simulink library "marine_gnc"  (Simulink 7.4)
settings: Solver=ode45  SolverMode=SingleTasking  StartTime=0.0  StopTime=10.0  RelTol=1e-3
undefined symbols (not defined in the file or in its folder): CN_data, CX_data, CY_data, D, G, K_supply, kt2ms, M, MA, magnitude, marine, Models, MRB, order, pathlength, RAO_Amp, RAO_Dir, RAO_Freq, RAO_Phase, RAO_Vel, RAO_yaw_back, RAO_yaw_quant, RAO_yaw_quantization_flag, rho_a, Semi, sub, T_supply, table, Tanker, vessel, Vessels
libraries: marine_gnc x64, simulink x39, cybersealib x1
(part 5 of 6)

== system marine_gnc/Utilities/Math Operations/[-inf inf] to [-pi pi] ==
  note: r
  note: x
  x [-inf inf] : Inport  OutDataType=sfix(16)  OutScaling=2^0
  Constant : Constant  Value=2*pi  OutDataType=sfix(16)  OutScaling=2^0
  Gain : Gain  Gain=pi  ParameterDataType=sfix(16)  ParameterScaling=2^0  OutDataType=sfix(16)  OutScaling=2^0  SaturateOnIntegerOverflow=on  OutDataTypeStr=Inherit: Same as input  ParamDataTypeStr=Inherit: Same as input
  Math Function : Math  Operator=rem  OutDataType=sfix(16)  OutScaling=2^0  SaturateOnIntegerOverflow=on
  Saturation : Saturate  UpperLimit=1e10  LowerLimit=-1e10
  Sign : Signum
  Sum : Sum  Inputs=|+-  OutDataType=sfix(16)  OutScaling=2^0  SaturateOnIntegerOverflow=on
  Sum1 : Sum  Inputs=|++  OutDataType=sfix(16)  OutScaling=2^0  SaturateOnIntegerOverflow=on
  y [-pi pi] : Outport  OutDataType=sfix(16)  OutScaling=2^0
  wires:
  Saturation/1 -> Sign/1, Sum1/1
  Sum/1 -> y [-pi pi]/1
  Math Function/1 -> Sum/1
  Constant/1 -> Math Function/2
  Sum1/1 -> Math Function/1
  Gain/1 -> Sum1/2, Sum/2
  Sign/1 -> Gain/1
  x [-inf inf]/1 -> Saturation/1

== system marine_gnc/Utilities/Math Operations/[-pi pi] to [-inf inf] ==
  x [-pi pi] : Inport  OutDataType=sfix(16)  OutScaling=2^0
  S-Function : S-Function  FunctionName=pipi2inf  EnableBusSupport=off
  y [-inf inf] : Outport  OutDataType=sfix(16)  OutScaling=2^0
  wires:
  S-Function/1 -> y [-inf inf]/1
  x [-pi pi]/1 -> S-Function/1

== system marine_gnc/Utilities/Math Operations/deg to 180/180 ==
  note: r
  note: x
  x (deg) : Inport  OutDataType=sfix(16)  OutScaling=2^0
  Constant : Constant  Value=2*180  OutDataType=sfix(16)  OutScaling=2^0
  Gain : Gain  Gain=180  ParameterDataType=sfix(16)  ParameterScaling=2^0  OutDataType=sfix(16)  OutScaling=2^0  SaturateOnIntegerOverflow=on  OutDataTypeStr=Inherit: Same as input  ParamDataTypeStr=Inherit: Same as input
  Math Function : Math  Operator=rem  OutDataType=sfix(16)  OutScaling=2^0  SaturateOnIntegerOverflow=on
  Saturation : Saturate  UpperLimit=1e10  LowerLimit=-1e10
  Sign : Signum
  Sum : Sum  Inputs=|+-  OutDataType=sfix(16)  OutScaling=2^0  SaturateOnIntegerOverflow=on
  Sum1 : Sum  Inputs=|++  OutDataType=sfix(16)  OutScaling=2^0  SaturateOnIntegerOverflow=on
  -180<y<180 : Outport  OutDataType=sfix(16)  OutScaling=2^0
  wires:
  Sum/1 -> -180<y<180/1
  Math Function/1 -> Sum/1
  Constant/1 -> Math Function/2
  Sum1/1 -> Math Function/1
  Gain/1 -> Sum1/2, Sum/2
  Sign/1 -> Gain/1
  x (deg)/1 -> Saturation/1
  Saturation/1 -> Sign/1, Sum1/1

== system marine_gnc/Utilities/Simulation tools/6DOF comparison ==
  In 1 : Inport  OutDataType=sfix(16)  OutScaling=2^0
  In 2 : Inport  Port=2  OutDataType=sfix(16)  OutScaling=2^0
  6DOF comparison : Scope  NumInputPorts=6
      settings: TimeRange=200  YMin=-0.2~-0.15~-0.5~-0.2~-0.02~-0.015  YMax=0.3~0.175~0.5~0.2~0.02~0.0175  MaxDataPoints=20000
  Demux1 : Demux  Outputs=6
  Demux2 : Demux  Outputs=6
  Mux{,1..5} (6 alike) : Mux  Inputs=2
  wires:
  Demux2/1 -> Mux/1  "surge"
  Demux1/1 -> Mux/2  "surge"
  Demux2/2 -> Mux1/1  "sway"
  Demux2/3 -> Mux2/1  "heave"
  Demux2/4 -> Mux3/1  "roll"
  Demux2/5 -> Mux4/1  "pitch"
  Demux2/6 -> Mux5/1  "yaw"
  Demux1/2 -> Mux1/2
  Demux1/3 -> Mux2/2
  Demux1/4 -> Mux3/2
  Demux1/5 -> Mux4/2
  Demux1/6 -> Mux5/2
  In 1/1 -> Demux2/1
  In 2/1 -> Demux1/1
  Mux/1 -> 6DOF comparison/1  "surge"
  Mux1/1 -> 6DOF comparison/2  "sway"
  Mux2/1 -> 6DOF comparison/3  "heave"
  Mux3/1 -> 6DOF comparison/4  "roll"
  Mux4/1 -> 6DOF comparison/5  "pitch"
  Mux5/1 -> 6DOF comparison/6  "yaw"

== system marine_gnc/Utilities/Simulation tools/Signal range error ==
  Signal : Inport  OutDataType=sfix(16)  OutScaling=2^0
  Add : Sum  OutDataType=sfix(16)  OutScaling=2^-10
  Constant : Constant  Value=Values  OutDataType=sfix(16)  OutScaling=2^0
  MinMax : MinMax  Function=max  OutDataType=sfix(16)  OutScaling=2^0
  MinMax1 : MinMax  Function=max  OutDataType=sfix(16)  OutScaling=2^0
  MinMax2 : MinMax  OutDataType=sfix(16)  OutScaling=2^0
  MinMax3 : MinMax  OutDataType=sfix(16)  OutScaling=2^0
  Saturation : Saturate  UpperLimit=1  LowerLimit=0
  Saturation1 : Saturate  UpperLimit=1  LowerLimit=0
  Sign : Signum
  Sign1 : Signum
  Stop simulation : marine_gnc/Utilities/Simulation tools/Stop simulation  message=message
  Subtract : Sum  Inputs=+-  OutDataType=sfix(16)  OutScaling=2^-10
  Subtract1 : Sum  Inputs=-+  OutDataType=sfix(16)  OutScaling=2^-10
  wires:
  Sign/1 -> Saturation/1
  Signal/1 -> MinMax/1, MinMax2/1
  Constant/1 -> MinMax1/1, MinMax3/1
  MinMax/1 -> Subtract/1
  MinMax1/1 -> Subtract/2
  Subtract/1 -> Sign/1
  Saturation/1 -> Add/1
  Add/1 -> Stop simulation/1
  Sign1/1 -> Saturation1/1
  Subtract1/1 -> Sign1/1
  MinMax2/1 -> Subtract1/1
  MinMax3/1 -> Subtract1/2
  Saturation1/1 -> Add/2

== system marine_gnc/Environment/Wind/Wind/Slowly-varying wind ==
  Enable : EnablePort
  Band-Limited White Noise : simulink/Sources/Band-Limited White Noise  Cov=Par_Wind_speed_noise_pow  Ts=Par_Wind_sample_time  seed=Par_Wind_speed_seed
  "Band-Limited White Noise " : simulink/Sources/Band-Limited White Noise  Cov=Par_Wind_angle_noise_pow  Ts=Par_Wind_sample_time  seed=Par_Wind_angle_seed
  Gain : Gain  Gain=1/Par_Wind_speed_T  ParameterDataType=sfix(16)  ParameterScaling=2^0  OutDataType=sfix(16)  OutScaling=2^0  SaturateOnIntegerOverflow=on  OutDataTypeStr=Inherit: Same as input  ParamDataTypeStr=Inherit: Same as input
  "Gain " : Gain  Gain=1/Par_Wind_angle_T  ParameterDataType=sfix(16)  ParameterScaling=2^0  OutDataType=sfix(16)  OutScaling=2^0  SaturateOnIntegerOverflow=on  OutDataTypeStr=Inherit: Same as input  ParamDataTypeStr=Inherit: Same as input
  Integrator : Integrator  LimitOutput=on  UpperSaturationLimit=Par_Wind_speed_rand_max  LowerSaturationLimit=-Par_Wind_speed_rand_max
  "Integrator " : Integrator  LimitOutput=on  UpperSaturationLimit=Par_Wind_angle_rand_max  LowerSaturationLimit=-Par_Wind_angle_rand_max
  Sum : Sum  Inputs=|+-  OutDataType=sfix(16)  OutScaling=2^0  SaturateOnIntegerOverflow=on  InputSameDT=on  OutDataTypeStr=Inherit: Same as first input
  "Sum       " : Sum  Inputs=|+-  OutDataType=sfix(16)  OutScaling=2^0  SaturateOnIntegerOverflow=on  InputSameDT=on  OutDataTypeStr=Inherit: Same as first input
  angle : Outport  OutDataType=sfix(16)  OutScaling=2^0  InitialOutput=0
  speed : Outport  Port=2  OutDataType=sfix(16)  OutScaling=2^0  InitialOutput=0
  wires:
  Band-Limited White Noise/1 -> Sum/1
  Integrator/1 -> Sum/2, speed/1
  Sum/1 -> Gain/1
  Gain/1 -> Integrator/1
  "Band-Limited White Noise "/1 -> "Sum       "/1
  "Integrator "/1 -> "Sum       "/2, angle/1
  "Sum       "/1 -> "Gain "/1
  "Gain "/1 -> "Integrator "/1

== system marine_gnc/Environment/Wind/Wind/Wind gust ==
  u10 : Inport  OutDataType=sfix(16)  OutScaling=2^0
  Enable : EnablePort
  Clock : Clock
      settings: Decimation=10
  Dot Product : simulink/Math Operations/Dot Product  InputSameDT=on  OutDataType=sfix(16)  OutScaling=2^-10  DoSatur=off
  Frequencies : Constant  Value=Par_Wind_minfreq:(Par_Wind_maxfreq - Par_Wind_minfreq)/(Par_Wind_nfreq-1):Par_Wind_maxfreq  OutDataType=sfix(16)  OutScaling=2^0
  Gain : Gain  Gain=2  ParameterDataType=sfix(16)  ParameterScaling=2^0  OutDataType=sfix(16)  OutScaling=2^0  SaturateOnIntegerOverflow=on  OutDataTypeStr=Inherit: Same as input  ParamDataTypeStr=Inherit: Same as input
  Gain1 : Gain  Gain=2*pi  ParameterDataType=sfix(16)  ParameterScaling=2^0  OutDataType=sfix(16)  OutScaling=2^0  SaturateOnIntegerOverflow=on  OutDataTypeStr=Inherit: Same as input  ParamDataTypeStr=Inherit: Same as input
  Harris spectrum : Subsystem
  Math Function1 : Math  Operator=sqrt  OutDataType=sfix(16)  OutScaling=2^0  SaturateOnIntegerOverflow=on
  Multiport Switch : MultiPortSwitch  Inputs=2  RndMeth=Nearest  SaturateOnIntegerOverflow=on
  NORSOK spectrum : Subsystem
  Phase generator : Subsystem
  Product1 : Product  OutDataType=sfix(16)  OutScaling=2^0  SaturateOnIntegerOverflow=on  OutDataTypeStr=Inherit: Same as first input
  Product2 : Product  OutDataType=sfix(16)  OutScaling=2^0  SaturateOnIntegerOverflow=on  OutDataTypeStr=Inherit: Same as first input
  Saturation : Saturate  UpperLimit=2  LowerLimit=1
  Spectrum type : Constant  Value=Par_Wind_spectrum_type  OutDataType=sfix(16)  OutScaling=2^0
  Sum : Sum  OutDataType=sfix(16)  OutScaling=2^0  SaturateOnIntegerOverflow=on
  Trigonometric Function : Trigonometry
  dfreq : Constant  Value=(Par_Wind_maxfreq - Par_Wind_minfreq)/(Par_Wind_nfreq -1)  OutDataType=sfix(16)  OutScaling=2^0
  Gust : Outport  OutDataType=sfix(16)  OutScaling=2^0  InitialOutput=0
  wires:
  Saturation/1 -> Multiport Switch/1
  Frequencies/1 -> Harris spectrum/1(Freqs), NORSOK spectrum/1(Freqs), Gain1/1
  u10/1 -> NORSOK spectrum/2(u10), Harris spectrum/2(u10)
  Gain/1 -> Product1/1
  dfreq/1 -> Product1/2
  Product1/1 -> Math Function1/1
  Multiport Switch/1 -> Gain/1
  Spectrum type/1 -> Saturation/1
  Harris spectrum/1(S) -> Multiport Switch/2
  NORSOK spectrum/1(S) -> Multiport Switch/3
  Gain1/1 -> Product2/1
  Clock/1 -> Product2/2, Phase generator/Trigger
  Product2/1 -> Sum/1  "wt"
  Phase generator/1(Phase) -> Sum/2
  Sum/1 -> Trigonometric Function/1
  Math Function1/1 -> Dot Product/1  "Amp"
  Trigonometric Function/1 -> Dot Product/2  "sin(wt + phase)"
  Dot Product/1 -> Gust/1

== system marine_gnc/Examples/Vessels/CyberShipII/saturation ==
  tau : Inport  OutDataType=sfix(16)  OutScaling=2^0
  Demux : Demux  Outputs=3
  Mux1 : Mux  Inputs=3
  Saturation : Saturate  UpperLimit=2  LowerLimit=-2
  Saturation1 : Saturate  UpperLimit=1.5  LowerLimit=-1.5
  Saturation2 : Saturate  UpperLimit=1.5  LowerLimit=-1.5
  sat_tau : Outport  OutDataType=sfix(16)  OutScaling=2^0
  wires:
  Mux1/1 -> sat_tau/1
  tau/1 -> Demux/1
  Demux/1 -> Saturation/1
  Demux/2 -> Saturation1/1
  Demux/3 -> Saturation2/1
  Saturation/1 -> Mux1/1
  Saturation1/1 -> Mux1/2
  Saturation2/1 -> Mux1/3

== system marine_gnc/Examples/Vessels/Mariner class cargo ship  (2nd -order)/Ship model ==
  note: heading
      | angle
  rudder angle : Inport  OutDataType=sfix(16)  OutScaling=2^0
  Integrator : Integrator
  Nomoto 2nd-order model : TransferFcn  Numerator=[K*T3 K]  Denominator=[T1*T2 (T1+T2) 1]
  heading angle : Outport  OutDataType=sfix(16)  OutScaling=2^0
  heading rate : Outport  Port=2  OutDataType=sfix(16)  OutScaling=2^0
  wires:
  rudder angle/1 -> Nomoto 2nd-order model/1
  Nomoto 2nd-order model/1 -> heading rate/1, Integrator/1  "heading rate"
  Integrator/1 -> heading angle/1

== system marine_gnc/Examples/Vessels/Tanker (1st-order)/Ship model ==
  note: heading
      | angle
  rudder angle : Inport  OutDataType=sfix(16)  OutScaling=2^0
  " Nomoto  time constant" : Gain  Gain=1/T_supply  ParameterDataType=sfix(16)  ParameterScaling=2^0  OutDataType=sfix(16)  OutScaling=2^0  SaturateOnIntegerOverflow=on  OutDataTypeStr=Inherit: Same as input  ParamDataTypeStr=Inherit: Same as input
  Integrator : Integrator
  Integrator1 : Integrator
  Nomoto gain constant : Gain  Gain=K_supply  ParameterDataType=sfix(16)  ParameterScaling=2^0  OutDataType=sfix(16)  OutScaling=2^0  SaturateOnIntegerOverflow=on  OutDataTypeStr=Inherit: Same as input  ParamDataTypeStr=Inherit: Same as input
  Sum : Sum  Inputs=|+-  OutDataType=sfix(16)  OutScaling=2^0  SaturateOnIntegerOverflow=on  InputSameDT=on  OutDataTypeStr=Inherit: Same as first input
  heading angle : Outport  OutDataType=sfix(16)  OutScaling=2^0
  heading rate : Outport  Port=2  OutDataType=sfix(16)  OutScaling=2^0
  wires:
  Integrator1/1 -> heading angle/1
  Integrator/1 -> Sum/2, Integrator1/1, heading rate/1  "heading  rate"
  Nomoto gain constant/1 -> Sum/1
  rudder angle/1 -> Nomoto gain constant/1
  Sum/1 -> " Nomoto  time constant"/1
  " Nomoto  time constant"/1 -> Integrator/1

== system marine_gnc/Examples/Vessels/Tanker (2nd-order)/Ship model ==
  note: heading
      | angle
  rudder angle : Inport  OutDataType=sfix(16)  OutScaling=2^0
  Integrator : Integrator
  Nomoto 2nd-order model : TransferFcn  Numerator=[K*T3 K]  Denominator=[T1*T2 (T1+T2) 1]
  heading angle : Outport  OutDataType=sfix(16)  OutScaling=2^0
  heading rate : Outport  Port=2  OutDataType=sfix(16)  OutScaling=2^0
  wires:
  rudder angle/1 -> Nomoto 2nd-order model/1
  Nomoto 2nd-order model/1 -> heading rate/1, Integrator/1  "heading rate"
  Integrator/1 -> heading angle/1

== system marine_gnc/Examples/Vessels/m-file examples/Container ship: L = 175 m ==
  u : Inport  OutDataType=sfix(16)  OutScaling=2^0
  xo : Inport  Port=2  OutDataType=sfix(16)  OutScaling=2^0
  Integrator : Integrator  InitialConditionSource=external  InitialCondition=[1 1]  UpperSaturationLimit=10  LowerSaturationLimit=-10
  Mux1 : Mux  Inputs=2
  m-file : MATLABFcn  MATLABFcn=feval(vessmodel,u(1:dimx_model),u(dimx_model+1:length(u)))  Output1D=off
  x : Outport  OutDataType=sfix(16)  OutScaling=2^0
  wires:
  xo/1 -> Integrator/2
  u/1 -> Mux1/2
  Mux1/1 -> m-file/1
  Integrator/1 -> x/1, Mux1/1
  m-file/1 -> Integrator/1

== system marine_gnc/Examples/Vessels/m-file examples/Deep submergence rescue vehicle ==
  u : Inport  OutDataType=sfix(16)  OutScaling=2^0
  xo : Inport  Port=2  OutDataType=sfix(16)  OutScaling=2^0
  Integrator : Integrator  InitialConditionSource=external  InitialCondition=[1 1]  UpperSaturationLimit=10  LowerSaturationLimit=-10
  Mux1 : Mux  Inputs=2
  m-file : MATLABFcn  MATLABFcn=feval(vessmodel,u(1:dimx_model),u(dimx_model+1:length(u)))  Output1D=off
  x : Outport  OutDataType=sfix(16)  OutScaling=2^0
  wires:
  xo/1 -> Integrator/2
  u/1 -> Mux1/2
  Mux1/1 -> m-file/1
  Integrator/1 -> x/1, Mux1/1
  m-file/1 -> Integrator/1

== system marine_gnc/Examples/Vessels/m-file examples/Large tanker: L = 304 m ==
  u : Inport  OutDataType=sfix(16)  OutScaling=2^0
  xo : Inport  Port=2  OutDataType=sfix(16)  OutScaling=2^0
  Integrator : Integrator  InitialConditionSource=external  InitialCondition=[1 1]  UpperSaturationLimit=10  LowerSaturationLimit=-10
  Mux1 : Mux  Inputs=2
  m-file : MATLABFcn  MATLABFcn=feval(vessmodel,u(1:dimx_model),u(dimx_model+1:length(u)))  Output1D=off
  x : Outport  OutDataType=sfix(16)  OutScaling=2^0
  wires:
  xo/1 -> Integrator/2
  u/1 -> Mux1/2
  Mux1/1 -> m-file/1
  Integrator/1 -> x/1, Mux1/1
  m-file/1 -> Integrator/1

== system marine_gnc/Examples/Vessels/m-file examples/Mariner class vessel: L = 160 m ==
  u : Inport  OutDataType=sfix(16)  OutScaling=2^0
  xo : Inport  Port=2  OutDataType=sfix(16)  OutScaling=2^0
  Integrator : Integrator  InitialConditionSource=external  InitialCondition=[1 1]  UpperSaturationLimit=10  LowerSaturationLimit=-10
  Mux1 : Mux  Inputs=2
  m-file : MATLABFcn  MATLABFcn=feval(vessmodel,u(1:dimx_model),u(dimx_model+1:length(u)))  Output1D=off
  x : Outport  OutDataType=sfix(16)  OutScaling=2^0
  wires:
  xo/1 -> Integrator/2
  u/1 -> Mux1/2
  Mux1/1 -> m-file/1
  Integrator/1 -> x/1, Mux1/1
  m-file/1 -> Integrator/1

== system marine_gnc/Examples/Vessels/m-file examples/Naval Postgraduate School AUV ==
  u : Inport  OutDataType=sfix(16)  OutScaling=2^0
  xo : Inport  Port=2  OutDataType=sfix(16)  OutScaling=2^0
  Integrator : Integrator  InitialConditionSource=external  InitialCondition=[1 1]  UpperSaturationLimit=10  LowerSaturationLimit=-10
  Mux1 : Mux  Inputs=2
  m-file : MATLABFcn  MATLABFcn=feval(vessmodel,u(1:dimx_model),u(dimx_model+1:length(u)))  Output1D=off
  x : Outport  OutDataType=sfix(16)  OutScaling=2^0
  wires:
  xo/1 -> Integrator/2
  u/1 -> Mux1/2
  Mux1/1 -> m-file/1
  Integrator/1 -> x/1, Mux1/1
  m-file/1 -> Integrator/1

== system marine_gnc/Guidance/Way-point guidance block/Stop vessel/Reached endpoint ==
  IfAction : ActionPort
  Constant : Constant  Value=0  OutDataType=sfix(16)  OutScaling=2^0
  Stop Simulation : Stop
  stop : Constant  Value=stop  OutDataType=sfix(16)  OutScaling=2^0
  zero : Outport  OutDataType=sfix(16)  OutScaling=2^0
  wires:
  Constant/1 -> zero/1
  stop/1 -> Stop Simulation/1

== system marine_gnc/Guidance/Way-point guidance block/Stop vessel/Still travelling ==
  IfAction : ActionPort
  Constant : Constant  OutDataType=sfix(16)  OutScaling=2^0
  one : Outport  OutDataType=sfix(16)  OutScaling=2^0
  wires:
  Constant/1 -> one/1

== system marine_gnc/Guidance/Way-point guidance block/Thetacomputation/5th order algorithm ==
  theta : Inport  OutDataType=sfix(16)  OutScaling=2^0
  IfAction : ActionPort
  Constant1 : Constant  OutDataType=sfix(16)  OutScaling=2^0
  Constant2 : Constant  OutDataType=sfix(16)  OutScaling=2^0
  Math Function : Math  Operator=mod  OutDataType=sfix(16)  OutScaling=2^0  SaturateOnIntegerOverflow=on
  Mux1 : Mux  Inputs=6
  Product{,1..3} (4 alike) : Product  OutDataType=sfix(16)  OutScaling=2^0  SaturateOnIntegerOverflow=on  InputSameDT=on  OutDataTypeStr=Inherit: Same as first input
  theta_vector : Outport  OutDataType=sfix(16)  OutScaling=2^0
  wires:
  Constant1/1 -> Math Function/2
  Math Function/1 -> Product/1, Product1/2, Product2/2, Product3/2, Mux1/5, Product/2
  theta/1 -> Math Function/1
  Product/1 -> Product1/1, Mux1/4  "t^2"
  Product1/1 -> Product2/1, Mux1/3  "t^3"
  Product2/1 -> Mux1/2, Product3/1  "t^4"
  Product3/1 -> Mux1/1
  Constant2/1 -> Mux1/6
  Mux1/1 -> theta_vector/1

== system marine_gnc/Guidance/Way-point guidance block/Thetacomputation/Cubic splines ==
  theta : Inport  OutDataType=sfix(16)  OutScaling=2^0
  IfAction : ActionPort
  Constant1 : Constant  OutDataType=sfix(16)  OutScaling=2^0
  Constant2 : Constant  Value=0  OutDataType=sfix(16)  OutScaling=2^0
  Mux1 : Mux  Inputs=6
  Product : Product  OutDataType=sfix(16)  OutScaling=2^0  SaturateOnIntegerOverflow=on  InputSameDT=on  OutDataTypeStr=Inherit: Same as first input
  Product1 : Product  OutDataType=sfix(16)  OutScaling=2^0  SaturateOnIntegerOverflow=on  InputSameDT=on  OutDataTypeStr=Inherit: Same as first input
  theta_vector : Outport  OutDataType=sfix(16)  OutScaling=2^0
  wires:
  theta/1 -> Product/1, Product/2, Product1/2, Mux1/3
  Product/1 -> Product1/1, Mux1/2  "t^2"
  Mux1/1 -> theta_vector/1
  Product1/1 -> Mux1/1  "t^3"
  Constant1/1 -> Mux1/4
  Constant2/1 -> Mux1/5, Mux1/6

== system marine_gnc/Guidance/Way-point guidance block/vs_calculations/vs_calc ==
  ud : Inport  OutDataType=sfix(16)  OutScaling=2^0
  xd_theta : Inport  Port=2  OutDataType=sfix(16)  OutScaling=2^0
  yd_theta : Inport  Port=3  OutDataType=sfix(16)  OutScaling=2^0
  Math Function : Math  Operator=square  OutDataType=sfix(16)  OutScaling=2^0  SaturateOnIntegerOverflow=on
  Math Function1 : Math  Operator=square  OutDataType=sfix(16)  OutScaling=2^0  SaturateOnIntegerOverflow=on
  Math Function2 : Math  Operator=sqrt  OutDataType=sfix(16)  OutScaling=2^0  SaturateOnIntegerOverflow=on
  Product : Product  Inputs=*/  OutDataType=sfix(16)  OutScaling=2^0  SaturateOnIntegerOverflow=on  InputSameDT=on  OutDataTypeStr=Inherit: Same as first input
  Sum : Sum  Inputs=|++  OutDataType=sfix(16)  OutScaling=2^0  SaturateOnIntegerOverflow=on  InputSameDT=on  OutDataTypeStr=Inherit: Same as first input
  vs : Outport  OutDataType=sfix(16)  OutScaling=2^0
  wires:
  Math Function/1 -> Sum/1
  Math Function1/1 -> Sum/2
  Sum/1 -> Math Function2/1
  Math Function2/1 -> Product/2
  xd_theta/1 -> Math Function/1
  ud/1 -> Product/1
  Product/1 -> vs/1  "vs"
  yd_theta/1 -> Math Function1/1

== system marine_gnc/Guidance/Way-point guidance block/vs_calculations/vs_t_calc ==
  xd_theta : Inport  OutDataType=sfix(16)  OutScaling=2^0
  yd_theta : Inport  Port=2  OutDataType=sfix(16)  OutScaling=2^0
  ud_dot : Inport  Port=3  OutDataType=sfix(16)  OutScaling=2^0
  Math Function3 : Math  Operator=square  OutDataType=sfix(16)  OutScaling=2^0  SaturateOnIntegerOverflow=on
  Math Function4 : Math  Operator=square  OutDataType=sfix(16)  OutScaling=2^0  SaturateOnIntegerOverflow=on
  Math Function5 : Math  Operator=sqrt  OutDataType=sfix(16)  OutScaling=2^0  SaturateOnIntegerOverflow=on
  Product7 : Product  Inputs=*/  OutDataType=sfix(16)  OutScaling=2^0  SaturateOnIntegerOverflow=on  InputSameDT=on  OutDataTypeStr=Inherit: Same as first input
  Sum3 : Sum  Inputs=|++  OutDataType=sfix(16)  OutScaling=2^0  SaturateOnIntegerOverflow=on  InputSameDT=on  OutDataTypeStr=Inherit: Same as first input
  vs_t : Outport  OutDataType=sfix(16)  OutScaling=2^0
  wires:
  xd_theta/1 -> Math Function3/1
  yd_theta/1 -> Math Function4/1
  Math Function3/1 -> Sum3/1
  Math Function4/1 -> Sum3/2
  Sum3/1 -> Math Function5/1
  Math Function5/1 -> Product7/2
  ud_dot/1 -> Product7/1
  Product7/1 -> vs_t/1

== system marine_gnc/Guidance/Way-point guidance block/vs_calculations/vs_theta_calc ==
  xd_theta : Inport  OutDataType=sfix(16)  OutScaling=2^0
  xd_theta_2 : Inport  Port=2  OutDataType=sfix(16)  OutScaling=2^0
  yd_theta : Inport  Port=3  OutDataType=sfix(16)  OutScaling=2^0
  yd_theta_2 : Inport  Port=4  OutDataType=sfix(16)  OutScaling=2^0
  ud : Inport  Port=5  OutDataType=sfix(16)  OutScaling=2^0
  Fcn1 : Fcn  Expr=u^(3/2)
  Gain1 : Gain  Gain=-1  ParameterDataType=sfix(16)  ParameterScaling=2^0  OutDataType=sfix(16)  OutScaling=2^0  SaturateOnIntegerOverflow=on  OutDataTypeStr=Inherit: Same as input  ParamDataTypeStr=Inherit: Same as input
  Math Function2 : Math  Operator=square  OutDataType=sfix(16)  OutScaling=2^0  SaturateOnIntegerOverflow=on
  Math Function3 : Math  Operator=square  OutDataType=sfix(16)  OutScaling=2^0  SaturateOnIntegerOverflow=on
  Product4 : Product  OutDataType=sfix(16)  OutScaling=2^0  SaturateOnIntegerOverflow=on  InputSameDT=on  OutDataTypeStr=Inherit: Same as first input
  Product5 : Product  OutDataType=sfix(16)  OutScaling=2^0  SaturateOnIntegerOverflow=on  InputSameDT=on  OutDataTypeStr=Inherit: Same as first input
  Product6 : Product  Inputs=/*  OutDataType=sfix(16)  OutScaling=2^0  SaturateOnIntegerOverflow=on  InputSameDT=on  OutDataTypeStr=Inherit: Same as first input
  Product7 : Product  OutDataType=sfix(16)  OutScaling=2^0  SaturateOnIntegerOverflow=on  InputSameDT=on  OutDataTypeStr=Inherit: Same as first input
  Sum2 : Sum  Inputs=|++  OutDataType=sfix(16)  OutScaling=2^0  SaturateOnIntegerOverflow=on  InputSameDT=on  OutDataTypeStr=Inherit: Same as first input
  Sum3 : Sum  Inputs=|++  OutDataType=sfix(16)  OutScaling=2^0  SaturateOnIntegerOverflow=on  InputSameDT=on  OutDataTypeStr=Inherit: Same as first input
  vs_theta : Outport  OutDataType=sfix(16)  OutScaling=2^0
  wires:
  xd_theta/1 -> Math Function2/1, Product4/1
  yd_theta/1 -> Math Function3/1, Product5/1
  Math Function2/1 -> Sum2/1
  Math Function3/1 -> Sum2/2
  Sum2/1 -> Fcn1/1
  xd_theta_2/1 -> Product4/2
  yd_theta_2/1 -> Product5/2
  Product4/1 -> Sum3/1
  Product5/1 -> Sum3/2
  Fcn1/1 -> Product6/1
  Sum3/1 -> Product6/2
  Product6/1 -> Gain1/1
  Gain1/1 -> Product7/1
  ud/1 -> Product7/2
  Product7/1 -> vs_theta/1

== system marine_gnc/Models/ Kinetics /Support/3 to 6 DOF ==
  In1 : Inport  OutDataType=sfix(16)  OutScaling=2^0
  Constant : Constant  Value=0  OutDataType=sfix(16)  OutScaling=2^0
  Mux1 : Mux  Inputs=2
  Selector : Selector  InputPortWidth=4  IndexOptions=Index vector (dialog)  Indices="[1 2  4 4 4 3]"  OutputSizes=1
  Out1 : Outport  OutDataType=sfix(16)  OutScaling=2^0
  wires:
  Selector/1 -> Out1/1
  In1/1 -> Mux1/1
  Constant/1 -> Mux1/2
  Mux1/1 -> Selector/1

== system marine_gnc/Models/ Kinetics /Support/4 to 6 DOF ==
  In1 : Inport  OutDataType=sfix(16)  OutScaling=2^0
  Constant : Constant  Value=0  OutDataType=sfix(16)  OutScaling=2^0
  Mux1 : Mux  Inputs=2
  Selector : Selector  InputPortWidth=5  IndexOptions=Index vector (dialog)  Indices="[1 2  5 3 5 4]"  OutputSizes=1
  Out1 : Outport  OutDataType=sfix(16)  OutScaling=2^0
  wires:
  Selector/1 -> Out1/1
  In1/1 -> Mux1/1
  Constant/1 -> Mux1/2
  Mux1/1 -> Selector/1

== system marine_gnc/Models/ Kinetics /Support/6 DOF Coriolis forces ==
  M : Inport  OutDataType=sfix(16)  OutScaling=2^0
  nu : Inport  Port=2  OutDataType=sfix(16)  OutScaling=2^0
  3x3 cross product : Subsystem
      mask Type: CrossProduct
      mask Description: Calculate the cross product of two 3-by-1 vectors.
      mask Display:
      | text(.5,.5,'Cross\nProduct\nc = axb', ...
      | 	'HorizontalAlignment','Center',...
      | 	'VerticalAlignment','middle')
  3x3 cross product1 : Subsystem
      mask Type: CrossProduct
      mask Description: Calculate the cross product of two 3-by-1 vectors.
      mask Display:
      | text(.5,.5,'Cross\nProduct\nc = axb', ...
      | 	'HorizontalAlignment','Center',...
      | 	'VerticalAlignment','middle')
  3x3 cross product2 : Subsystem
      mask Type: CrossProduct
      mask Description: Calculate the cross product of two 3-by-1 vectors.
      mask Display:
      | text(.5,.5,'Cross\nProduct\nc = axb', ...
      | 	'HorizontalAlignment','Center',...
      | 	'VerticalAlignment','middle')
  Gain : Gain  Gain=0.5  ParameterDataType=sfix(16)  ParameterScaling=2^0  OutDataType=sfix(16)  OutScaling=2^0  SaturateOnIntegerOverflow=on  OutDataTypeStr=Inherit: Same as input  ParamDataTypeStr=Inherit: Same as input
  Gain1 : Gain  Gain=-1  ParameterDataType=sfix(16)  ParameterScaling=2^0  OutDataType=sfix(16)  OutScaling=2^0  SaturateOnIntegerOverflow=on  OutDataTypeStr=Inherit: Same as input  ParamDataTypeStr=Inherit: Same as input
  Gain2 : Gain  Gain=-1  ParameterDataType=sfix(16)  ParameterScaling=2^0  OutDataType=sfix(16)  OutScaling=2^0  SaturateOnIntegerOverflow=on  OutDataTypeStr=Inherit: Same as input  ParamDataTypeStr=Inherit: Same as input
  M11 : Selector  NumberOfDimensions=2  InputPortWidth=3  IndexOptions=Index vector (dialog),Index vector (dialog)  Indices=[1 2 3],[1 2 3]  OutputSizes=1
  M12 : Selector  NumberOfDimensions=2  InputPortWidth=3  IndexOptions=Index vector (dialog),Index vector (dialog)  Indices=[1 2 3],[4 5 6]  OutputSizes=1
  M22 : Selector  NumberOfDimensions=2  InputPortWidth=3  IndexOptions=Index vector (dialog),Index vector (dialog)  Indices=[4 5 6],[4 5 6]  OutputSizes=1
  Mux : Mux  Inputs=2
  Product{,1..3} (4 alike) : Product  Multiplication=Matrix(*)  OutDataType=sfix(16)  OutScaling=2^0  SaturateOnIntegerOverflow=on  OutDataTypeStr=Inherit: Same as first input
  Selector : Selector  InputPortWidth=6  IndexOptions=Index vector (dialog)  Indices=[1 2 3]  OutputSizes=1
  Selector1 : Selector  InputPortWidth=6  IndexOptions=Index vector (dialog)  Indices=[4 5 6]  OutputSizes=1
  Sum{,1..3} (4 alike) : Sum  Inputs=|++  OutDataType=sfix(16)  OutScaling=2^0  SaturateOnIntegerOverflow=on
  transpose : Math  Operator=transpose  OutDataType=sfix(16)  OutScaling=2^0  SaturateOnIntegerOverflow=on
  transpose1 : Math  Operator=transpose  OutDataType=sfix(16)  OutScaling=2^0  SaturateOnIntegerOverflow=on
  C(nu)nu : Outport  OutDataType=sfix(16)  OutScaling=2^0
  wires:
  M/1 -> Sum/1, transpose/1  "M"
  nu/1 -> Selector1/1, Selector/1
  Mux/1 -> C(nu)nu/1  "C(nu)nu"
  Sum3/1 -> Mux/2
  3x3 cross product2/1(c) -> Sum3/2
  3x3 cross product1/1(c) -> Sum3/1
  Gain2/1 -> 3x3 cross product2/1(a)
  3x3 cross product/1(c) -> Mux/1
  Gain1/1 -> 3x3 cross product/1(a), 3x3 cross product1/1(a)
  Sum2/1 -> Gain2/1  "dT/d(nu2)"
  Product3/1 -> Sum2/2  "M22*nu2"
  M22/1 -> Product3/1
  Product2/1 -> Sum2/1  "M21*nu1"
  transpose1/1 -> Product2/1  "M21=M12'"
  Sum1/1 -> Gain1/1  "dT/d(nu1)"
  Product1/1 -> Sum1/2  "M12*nu2"
  M12/1 -> Product1/1, transpose1/1
  Product/1 -> Sum1/1  "M11*nu1"
  M11/1 -> Product/1
  Selector1/1 -> Product1/2, Product3/2, 3x3 cross product/2(b), 3x3 cross product2/2(b)  "nu2"
  Selector/1 -> Product/2, Product2/2, 3x3 cross product1/2(b)  "nu1"
  Gain/1 -> M11/1, M12/1, M22/1  "1/2 (M+M')"
  Sum/1 -> Gain/1
  transpose/1 -> Sum/2  "M'"

== system marine_gnc/Models/ Kinetics /Support/M33 to M66 ==
  M33 : Inport  OutDataType=sfix(16)  OutScaling=2^0
  Product : Product  Inputs=3  Multiplication=Matrix(*)  OutDataType=sfix(16)  OutScaling=2^0  SaturateOnIntegerOverflow=on  OutDataTypeStr=Inherit: Same as first input
  modes : Constant  Value=[1 0 0; 0 1 0; 0 0 0; 0 0 0; 0 0 0; 0 0 1]  OutDataType=sfix(16)  OutScaling=2^0
  transpose : Math  Operator=transpose  OutDataType=sfix(16)  OutScaling=2^0  SaturateOnIntegerOverflow=on
  M66 : Outport  OutDataType=sfix(16)  OutScaling=2^0
  wires:
  modes/1 -> transpose/1, Product/1
  transpose/1 -> Product/3
  M33/1 -> Product/2
  Product/1 -> M66/1

== system marine_gnc/Models/ Kinetics /Support/M44 to M66 ==
  M44 : Inport  OutDataType=sfix(16)  OutScaling=2^0
  Product : Product  Inputs=3  Multiplication=Matrix(*)  OutDataType=sfix(16)  OutScaling=2^0  SaturateOnIntegerOverflow=on  OutDataTypeStr=Inherit: Same as first input
  modes : Constant  Value=[1 0 0 0; 0 1 0 0; 0 0 0 0; 0 0 1 0; 0 0 0 0; 0 0 0 1]  OutDataType=sfix(16)  OutScaling=2^0
  transpose : Math  Operator=transpose  OutDataType=sfix(16)  OutScaling=2^0  SaturateOnIntegerOverflow=on
  M66 : Outport  OutDataType=sfix(16)  OutScaling=2^0
  wires:
  modes/1 -> transpose/1, Product/1
  transpose/1 -> Product/3
  M44/1 -> Product/2
  Product/1 -> M66/1

== system marine_gnc/Models/Environmental Loads/Force RAO/Wave component loop ==
  number of  iterations : Inport  OutDataType=sfix(16)  OutScaling=2^0
  Psi_r : Inport  Port=2  OutDataType=sfix(16)  OutScaling=2^0
  Omega : Inport  Port=3  OutDataType=sfix(16)  OutScaling=2^0
  Phase_tot : Inport  Port=4  OutDataType=sfix(16)  OutScaling=2^0
  Zeta_a : Inport  Port=5  OutDataType=sfix(16)  OutScaling=2^0
  U : Inport  Port=6  OutDataType=sfix(16)  OutScaling=2^0
  "                " : Trigonometry
  "                1" : Trigonometry  Operator=cos
  For Iterator : ForIterator  ResetStates=reset  IterationSource=external  IterationVariableDataType=double
  Memory1 : Memory  X0=[0 0 0 0 0 0]'  InheritSampleTime=on
  Memory2 : Memory  X0=[0 0 0 0 0 0]'  InheritSampleTime=on
  Product1 : Product  OutDataType=sfix(16)  OutScaling=2^0  SaturateOnIntegerOverflow=on  OutDataTypeStr=Inherit: Same as first input
  Product3 : Product  Inputs=3  OutDataType=sfix(16)  OutScaling=2^0  SaturateOnIntegerOverflow=on  OutDataTypeStr=Inherit: Same as first input
  Product4 : Product  OutDataType=sfix(16)  OutScaling=2^0  SaturateOnIntegerOverflow=on  OutDataTypeStr=Inherit: Same as first input
  RAO tables : marine_gnc/Models/Environmental Loads/Utilities/RAO tables  RAO_Freq=RAO_Freq  RAO_Dir=RAO_Dir  RAO_Vel=RAO_Vel  RAO_Amp=RAO_Amp  RAO_Phase=RAO_Phase
  Selector{2..5} (4 alike) : Selector  IndexOptions=Index vector (port)  Indices=[1 3]  OutputSizes=1
  Sum1 : Sum  Inputs=++|  OutDataType=sfix(16)  OutScaling=2^0  SaturateOnIntegerOverflow=on
  Sum4 : Sum  Inputs=++|  OutDataType=sfix(16)  OutScaling=2^0  SaturateOnIntegerOverflow=on
  Sum5 : Sum  Inputs=++|  OutDataType=sfix(16)  OutScaling=2^0  SaturateOnIntegerOverflow=on
  Tau WF : Outport  OutDataType=sfix(16)  OutScaling=2^0
  Tau rate : Outport  Port=2  OutDataType=sfix(16)  OutScaling=2^0
  wires:
  "                1"/1 -> Product3/1
  Sum1/1 -> Memory1/1, Tau rate/1
  Memory1/1 -> Sum1/2
  Product3/1 -> Sum1/1
  Product4/1 -> Product3/2, Product1/2
  "                "/1 -> Product1/1
  Selector3/1 -> RAO tables/1  "psi_r"
  Selector2/1 -> Product3/3, RAO tables/2  "omega"
  Selector5/1 -> Sum5/2  "phase"
  Product1/1 -> Sum4/1
  Memory2/1 -> Sum4/2
  Sum4/1 -> Tau WF/1, Memory2/1
  number of  iterations/1 -> For Iterator/1
  Omega/1 -> Selector2/1
  For Iterator/1 -> Selector4/2, Selector5/2, Selector2/2, Selector3/2  "i=1:N"
  Psi_r/1 -> Selector3/1
  U/1 -> RAO tables/3
  RAO tables/1 -> Product4/1
  RAO tables/2 -> Sum5/1
  Phase_tot/1 -> Selector5/1
  Zeta_a/1 -> Selector4/1
  Sum5/1 -> "                1"/1, "                "/1
  Selector4/1 -> Product4/2  "zeta_a"

== system marine_gnc/Models/Environmental Loads/Isherwood (1972) wind data/If gamm_r > 0  then feedthrough ==
  6 DOF : Inport  OutDataType=sfix(16)  OutScaling=2^0
  Action Port : ActionPort
  "6 DOF  " : Outport  OutDataType=sfix(16)  OutScaling=2^0
  wires:
  6 DOF/1 -> "6 DOF  "/1

== system marine_gnc/Models/Environmental Loads/Isherwood (1972) wind data/If gamma_r <0 then change sign ==
  6 DOF : Inport  OutDataType=sfix(16)  OutScaling=2^0
  Action Port : ActionPort
  Constant : Constant  Value=[1 -1 1 -1 1 -1]  OutDataType=sfix(16)  OutScaling=2^0
  Product : Product  OutDataType=sfix(16)  OutScaling=2^0  SaturateOnIntegerOverflow=on  OutDataTypeStr=Inherit: Same as first input
  "6 DOF  " : Outport  OutDataType=sfix(16)  OutScaling=2^0
  wires:
  Constant/1 -> Product/2
  Product/1 -> "6 DOF  "/1
  6 DOF/1 -> Product/1

== system marine_gnc/Models/Environmental Loads/Motion RAO/6DOF rotation matrix in yaw ==
  psi : Inport  OutDataType=sfix(16)  OutScaling=2^0
  V : Inport  Port=2  OutDataType=sfix(16)  OutScaling=2^0
  Mux1 : Mux  Inputs=2
  Rotation matrix in yaw : marine_gnc/Models/ Kinematics/Rotation matrix in yaw 
  Selector : Selector  InputPortWidth=6  IndexOptions=Index vector (dialog)  Indices=[4 5 6]  OutputSizes=1
  Selector2 : Selector  InputPortWidth=6  IndexOptions=Index vector (dialog)  Indices=[1 2 3]  OutputSizes=1
  R(psi)*V : Outport  OutDataType=sfix(16)  OutScaling=2^0
  wires:
  Rotation matrix in yaw/1 -> Mux1/1
  V/1 -> Selector/1, Selector2/1
  psi/1 -> Rotation matrix in yaw/1
  Selector2/1 -> Rotation matrix in yaw/2
  Mux1/1 -> R(psi)*V/1
  Selector/1 -> Mux1/2

== system marine_gnc/Models/Environmental Loads/Motion RAO/Output smoothing ==
  eta_h WF : Inport  OutDataType=sfix(16)  OutScaling=2^0
  "nu WF " : Inport  Port=2  OutDataType=sfix(16)  OutScaling=2^0
  "nu_dot WF " : Inport  Port=3  OutDataType=sfix(16)  OutScaling=2^0
  nu_dot rate : Inport  Port=4  OutDataType=sfix(16)  OutScaling=2^0
  Output smoothing flag : Constant  Value=RAO_smoothing_flag  OutDataType=sfix(16)  OutScaling=2^0
  Signal smoothing : marine_gnc/Models/Environmental Loads/Utilities/Signal smoothing
  Signal smoothing1 : marine_gnc/Models/Environmental Loads/Utilities/Signal smoothing
  Signal smoothing2 : marine_gnc/Models/Environmental Loads/Utilities/Signal smoothing
  Switch1 : Switch  Threshold=0.5
  Switch2 : Switch  Threshold=0.5
  Switch3 : Switch  Threshold=0.5
  "eta_h WF " : Outport  OutDataType=sfix(16)  OutScaling=2^0
  nu WF : Outport  Port=2  OutDataType=sfix(16)  OutScaling=2^0
  nu_dot WF : Outport  Port=3  OutDataType=sfix(16)  OutScaling=2^0
  wires:
  Switch1/1 -> nu WF/1
  Switch3/1 -> nu_dot WF/1
  nu_dot rate/1 -> Signal smoothing2/2
  Signal smoothing2/1 -> Switch3/1
  "nu_dot WF "/1 -> Switch3/3, Signal smoothing1/2, Signal smoothing2/1
  Switch2/1 -> "eta_h WF "/1
  Signal smoothing1/1 -> Switch1/1
  "nu WF "/1 -> Switch1/3, Signal smoothing/2, Signal smoothing1/1
  eta_h WF/1 -> Switch2/3, Signal smoothing/1
  Signal smoothing/1 -> Switch2/1
  Output smoothing flag/1 -> Switch3/2, Switch1/2, Switch2/2

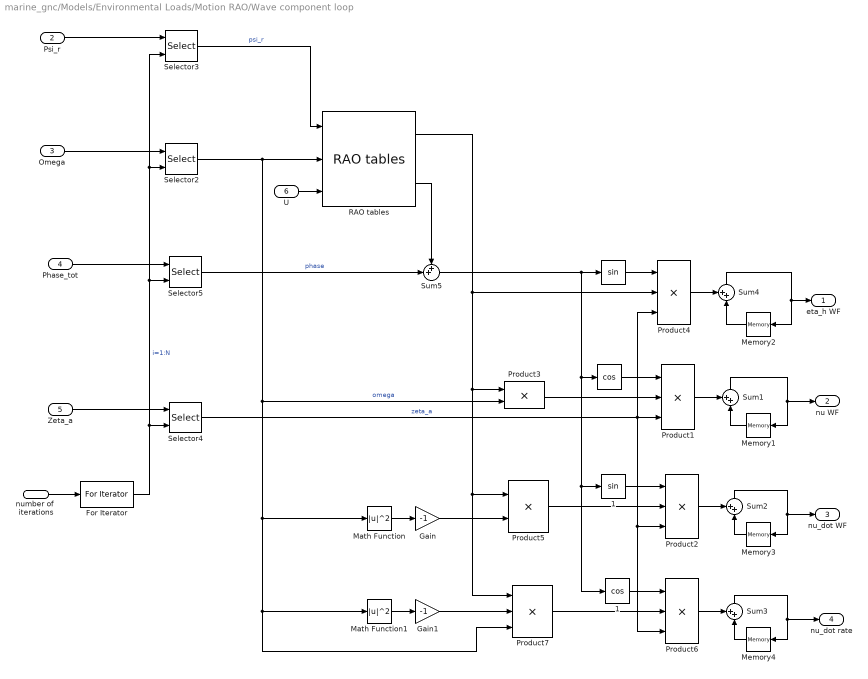
== system marine_gnc/Models/Environmental Loads/Motion RAO/Wave component loop ==
  number of  iterations : Inport  OutDataType=sfix(16)  OutScaling=2^0
  Psi_r : Inport  Port=2  OutDataType=sfix(16)  OutScaling=2^0
  Omega : Inport  Port=3  OutDataType=sfix(16)  OutScaling=2^0
  Phase_tot : Inport  Port=4  OutDataType=sfix(16)  OutScaling=2^0
  Zeta_a : Inport  Port=5  OutDataType=sfix(16)  OutScaling=2^0
  U : Inport  Port=6  OutDataType=sfix(16)  OutScaling=2^0
  "              " : Trigonometry  Operator=cos
  "                " : Trigonometry
  "                1" : Trigonometry
  "              1" : Trigonometry  Operator=cos
  For Iterator : ForIterator  ResetStates=reset  IterationSource=external  IterationVariableDataType=double
  Gain : Gain  Gain=-1  ParameterDataType=sfix(16)  ParameterScaling=2^0  OutDataType=sfix(16)  OutScaling=2^0  SaturateOnIntegerOverflow=on  OutDataTypeStr=Inherit: Same as input  ParamDataTypeStr=Inherit: Same as input
  Gain1 : Gain  Gain=-1  ParameterDataType=sfix(16)  ParameterScaling=2^0  OutDataType=sfix(16)  OutScaling=2^0  SaturateOnIntegerOverflow=on  OutDataTypeStr=Inherit: Same as input  ParamDataTypeStr=Inherit: Same as input
  Math Function : Math  Operator=magnitude^2  OutDataType=sfix(16)  OutScaling=2^0  SaturateOnIntegerOverflow=on
  Math Function1 : Math  Operator=magnitude^2  OutDataType=sfix(16)  OutScaling=2^0  SaturateOnIntegerOverflow=on
  Memory{1..4} (4 alike) : Memory  X0=[0 0 0 0 0 0]'  InheritSampleTime=on
  Product{1..2,4,6} (4 alike) : Product  Inputs=3  OutDataType=sfix(16)  OutScaling=2^0  SaturateOnIntegerOverflow=on  OutDataTypeStr=Inherit: Same as first input
  Product3 : Product  Inputs=**  OutDataType=sfix(16)  OutScaling=2^0  SaturateOnIntegerOverflow=on  OutDataTypeStr=Inherit: Same as first input
  Product5 : Product  Inputs=**  OutDataType=sfix(16)  OutScaling=2^0  SaturateOnIntegerOverflow=on  OutDataTypeStr=Inherit: Same as first input
  Product7 : Product  Inputs=***  OutDataType=sfix(16)  OutScaling=2^0  SaturateOnIntegerOverflow=on  OutDataTypeStr=Inherit: Same as first input
  RAO tables : marine_gnc/Models/Environmental Loads/Utilities/RAO tables  RAO_Freq=RAO_Freq  RAO_Dir=RAO_Dir  RAO_Vel=RAO_Vel  RAO_Amp=RAO_Amp  RAO_Phase=RAO_Phase
  Selector{2..5} (4 alike) : Selector  IndexOptions=Index vector (port)  Indices=[1 3]  OutputSizes=1
  Sum{1..5} (5 alike) : Sum  Inputs=++|  OutDataType=sfix(16)  OutScaling=2^0  SaturateOnIntegerOverflow=on
  eta_h WF : Outport  OutDataType=sfix(16)  OutScaling=2^0
  nu WF : Outport  Port=2  OutDataType=sfix(16)  OutScaling=2^0
  nu_dot WF : Outport  Port=3  OutDataType=sfix(16)  OutScaling=2^0
  nu_dot rate : Outport  Port=4  OutDataType=sfix(16)  OutScaling=2^0
  wires:
  Product7/1 -> Product6/2
  "              1"/1 -> Product6/1
  Math Function1/1 -> Gain1/1
  Gain1/1 -> Product7/2
  Memory4/1 -> Sum3/2
  Product6/1 -> Sum3/1
  Sum3/1 -> Memory4/1, nu_dot rate/1
  Selector3/1 -> RAO tables/1  "psi_r"
  Selector2/1 -> Product7/3, Math Function1/1, Math Function/1, Product3/2, RAO tables/2  "omega"
  Selector5/1 -> Sum5/2  "phase"
  Product4/1 -> Sum4/1
  Memory2/1 -> Sum4/2
  Sum4/1 -> eta_h WF/1, Memory2/1
  number of  iterations/1 -> For Iterator/1
  Omega/1 -> Selector2/1
  For Iterator/1 -> Selector3/2, Selector2/2, Selector5/2, Selector4/2  "i=1:N"
  Psi_r/1 -> Selector3/1
  U/1 -> RAO tables/3
  RAO tables/1 -> Product4/2, Product7/1, Product5/1, Product3/1
  RAO tables/2 -> Sum5/1
  Phase_tot/1 -> Selector5/1
  Zeta_a/1 -> Selector4/1
  Sum5/1 -> "                "/1, "              1"/1, "                1"/1, "              "/1
  "                "/1 -> Product4/1
  Selector4/1 -> Product6/3, Product2/3, Product1/3, Product4/3  "zeta_a"
  "              "/1 -> Product1/1
  Memory1/1 -> Sum1/2
  Sum1/1 -> nu WF/1, Memory1/1
  Product1/1 -> Sum1/1
  Memory3/1 -> Sum2/2
  Product2/1 -> Sum2/1
  Sum2/1 -> nu_dot WF/1, Memory3/1
  "                1"/1 -> Product2/1
  Math Function/1 -> Gain/1
  Gain/1 -> Product5/2
  Product5/1 -> Product2/2
  Product3/1 -> Product1/2

== system marine_gnc/Models/Environmental Loads/Utilities/Position phase ==
  psi wave : Inport  OutDataType=sfix(16)  OutScaling=2^0
  wavenum : Inport  Port=2  OutDataType=sfix(16)  OutScaling=2^0
  eta LF : Inport  Port=3  OutDataType=sfix(16)  OutScaling=2^0
  Product2 : Product  Inputs=**  OutDataType=sfix(16)  OutScaling=2^0  SaturateOnIntegerOverflow=on  OutDataTypeStr=Inherit: Same as first input
  Product6 : Product  Inputs=**  OutDataType=sfix(16)  OutScaling=2^0  SaturateOnIntegerOverflow=on  OutDataTypeStr=Inherit: Same as first input
  Product7 : Product  Inputs=**  OutDataType=sfix(16)  OutScaling=2^0  SaturateOnIntegerOverflow=on  OutDataTypeStr=Inherit: Same as first input
  Sum5 : Sum  OutDataType=sfix(16)  OutScaling=2^0  SaturateOnIntegerOverflow=on
  cos : Trigonometry  Operator=cos
  sin : Trigonometry
  x-position : Selector  IndexOptions=Index vector (dialog)  Indices=1  OutputSizes=1
  y-position : Selector  InputPortWidth=6  IndexOptions=Index vector (dialog)  Indices=2  OutputSizes=1
  pos phase : Outport  OutDataType=sfix(16)  OutScaling=2^0
  wires:
  wavenum/1 -> Product7/2
  Product7/1 -> pos phase/1
  eta LF/1 -> y-position/1, x-position/1
  psi wave/1 -> cos/1, sin/1
  Product6/1 -> Sum5/2
  y-position/1 -> Product2/2
  x-position/1 -> Product6/2
  cos/1 -> Product6/1
  sin/1 -> Product2/1
  Product2/1 -> Sum5/1
  Sum5/1 -> Product7/1

== system marine_gnc/Models/Environmental Loads/Utilities/RAO tables ==
  psi_r : Inport  OutDataType=sfix(16)  OutScaling=2^0
  omega : Inport  Port=2  OutDataType=sfix(16)  OutScaling=2^0
  U : Inport  Port=3  OutDataType=sfix(16)  OutScaling=2^0
  Abs : Abs  SaturateOnIntegerOverflow=on
  Amplitude table lookup1 : simulink/Lookup Tables/Lookup Table (n-D)  numDimsPopupSelect=3  bp1=RAO_Freq  bp2=RAO_Dir  bp3=RAO_Vel  bp4=[1:3]  bpcell={ [1:3], [1:3] }  explicitNumDims=2  searchMode=Binary Search  cacheBpFlag=off  vectorInputFlag=off  tableData=RAO_Amp{1}  interpMethod=Linear  extrapMethod=Linear  rangeErrorMode=Warning
  Amplitude table lookup2 : simulink/Lookup Tables/Lookup Table (n-D)  numDimsPopupSelect=3  bp1=RAO_Freq  bp2=RAO_Dir  bp3=RAO_Vel  bp4=[1:3]  bpcell={ [1:3], [1:3] }  explicitNumDims=2  searchMode=Binary Search  cacheBpFlag=off  vectorInputFlag=off  tableData=RAO_Amp{2}  interpMethod=Linear  extrapMethod=Linear  rangeErrorMode=None
  Amplitude table lookup3 : simulink/Lookup Tables/Lookup Table (n-D)  numDimsPopupSelect=3  bp1=RAO_Freq  bp2=RAO_Dir  bp3=RAO_Vel  bp4=[1:3]  bpcell={ [1:3], [1:3] }  explicitNumDims=2  searchMode=Binary Search  cacheBpFlag=off  vectorInputFlag=off  tableData=RAO_Amp{3}  interpMethod=Linear  extrapMethod=Linear  rangeErrorMode=None
  Amplitude table lookup4 : simulink/Lookup Tables/Lookup Table (n-D)  numDimsPopupSelect=3  bp1=RAO_Freq  bp2=RAO_Dir  bp3=RAO_Vel  bp4=[1:3]  bpcell={ [1:3], [1:3] }  explicitNumDims=2  searchMode=Binary Search  cacheBpFlag=off  vectorInputFlag=off  tableData=RAO_Amp{4}  interpMethod=Linear  extrapMethod=Linear  rangeErrorMode=None
  Amplitude table lookup5 : simulink/Lookup Tables/Lookup Table (n-D)  numDimsPopupSelect=3  bp1=RAO_Freq  bp2=RAO_Dir  bp3=RAO_Vel  bp4=[1:3]  bpcell={ [1:3], [1:3] }  explicitNumDims=2  searchMode=Binary Search  cacheBpFlag=off  vectorInputFlag=off  tableData=RAO_Amp {5}  interpMethod=Linear  extrapMethod=Linear  rangeErrorMode=None
  Amplitude table lookup6 : simulink/Lookup Tables/Lookup Table (n-D)  numDimsPopupSelect=3  bp1=RAO_Freq  bp2=RAO_Dir  bp3=RAO_Vel  bp4=[1:3]  bpcell={ [1:3], [1:3] }  explicitNumDims=2  searchMode=Binary Search  cacheBpFlag=off  vectorInputFlag=off  tableData=RAO_Amp{6}  interpMethod=Linear  extrapMethod=Linear  rangeErrorMode=None
  Mux1 : Mux  Inputs=6
  Mux2 : Mux  Inputs=6
  Phase table lookup1 : simulink/Lookup Tables/Lookup Table (n-D)  numDimsPopupSelect=3  bp1=RAO_Freq  bp2=RAO_Dir  bp3=RAO_Vel  bp4=[1:3]  bpcell={ [1:3], [1:3] }  explicitNumDims=2  searchMode=Binary Search  cacheBpFlag=off  vectorInputFlag=off  tableData=RAO_Phase{1}  interpMethod=Linear  extrapMethod=Linear  rangeErrorMode=None
  Phase table lookup2 : simulink/Lookup Tables/Lookup Table (n-D)  numDimsPopupSelect=3  bp1=RAO_Freq  bp2=RAO_Dir  bp3=RAO_Vel  bp4=[1:3]  bpcell={ [1:3], [1:3] }  explicitNumDims=2  searchMode=Binary Search  cacheBpFlag=off  vectorInputFlag=off  tableData=RAO_Phase{2}  interpMethod=Linear  extrapMethod=Linear  rangeErrorMode=None
  Phase table lookup3 : simulink/Lookup Tables/Lookup Table (n-D)  numDimsPopupSelect=3  bp1=RAO_Freq  bp2=RAO_Dir  bp3=RAO_Vel  bp4=[1:3]  bpcell={ [1:3], [1:3] }  explicitNumDims=2  searchMode=Binary Search  cacheBpFlag=off  vectorInputFlag=off  tableData=RAO_Phase{3}  interpMethod=Linear  extrapMethod=Linear  rangeErrorMode=None
  Phase table lookup4 : simulink/Lookup Tables/Lookup Table (n-D)  numDimsPopupSelect=3  bp1=RAO_Freq  bp2=RAO_Dir  bp3=RAO_Vel  bp4=[1:3]  bpcell={ [1:3], [1:3] }  explicitNumDims=2  searchMode=Binary Search  cacheBpFlag=off  vectorInputFlag=off  tableData=RAO_Phase{4}  interpMethod=Linear  extrapMethod=Linear  rangeErrorMode=None
  Phase table lookup5 : simulink/Lookup Tables/Lookup Table (n-D)  numDimsPopupSelect=3  bp1=RAO_Freq  bp2=RAO_Dir  bp3=RAO_Vel  bp4=[1:3]  bpcell={ [1:3], [1:3] }  explicitNumDims=2  searchMode=Binary Search  cacheBpFlag=off  vectorInputFlag=off  tableData=RAO_Phase{5}  interpMethod=Linear  extrapMethod=Linear  rangeErrorMode=None
  Phase table lookup6 : simulink/Lookup Tables/Lookup Table (n-D)  numDimsPopupSelect=3  bp1=RAO_Freq  bp2=RAO_Dir  bp3=RAO_Vel  bp4=[1:3]  bpcell={ [1:3], [1:3] }  explicitNumDims=2  searchMode=Binary Search  cacheBpFlag=off  vectorInputFlag=off  tableData=RAO_Phase{6}  interpMethod=Linear  extrapMethod=Linear  rangeErrorMode=None
  Product1 : Product  Inputs=**  OutDataType=sfix(16)  OutScaling=2^0  SaturateOnIntegerOverflow=on  OutDataTypeStr=Inherit: Same as first input
  Product2 : Product  Inputs=**  OutDataType=sfix(16)  OutScaling=2^0  SaturateOnIntegerOverflow=on  OutDataTypeStr=Inherit: Same as first input
  Product3 : Product  Inputs=**  OutDataType=sfix(16)  OutScaling=2^0  SaturateOnIntegerOverflow=on  OutDataTypeStr=Inherit: Same as first input
  Sign : Signum
  "[-inf inf] to [-pi pi]" : marine_gnc/Utilities/Math Operations/[-inf inf] to [-pi pi]
  amp : Outport  OutDataType=sfix(16)  OutScaling=2^0
  phase : Outport  Port=2  OutDataType=sfix(16)  OutScaling=2^0
  wires:
  Amplitude table lookup1/1 -> Mux1/1
  omega/1 -> Amplitude table lookup1/1, Phase table lookup1/1, Phase table lookup5/1, Phase table lookup6/1, Phase table lookup4/1, Phase table lookup3/1, Phase table lookup2/1, Amplitude table lookup6/1, Amplitude table lookup5/1, Amplitude table lookup4/1, Amplitude table lookup3/1, Amplitude table lookup2/1
  "[-inf inf] to [-pi pi]"/1 -> Abs/1, Sign/1
  Amplitude table lookup3/1 -> Mux1/3
  Amplitude table lookup5/1 -> Mux1/5
  Abs/1 -> Amplitude table lookup1/2, Phase table lookup1/2, Phase table lookup5/2, Phase table lookup6/2, Phase table lookup4/2, Phase table lookup3/2, Phase table lookup2/2, Amplitude table lookup6/2, Amplitude table lookup5/2, Amplitude table lookup4/2, Amplitude table lookup3/2, Amplitude table lookup2/2
  Product1/1 -> Mux1/2
  Amplitude table lookup2/1 -> Product1/2
  Sign/1 -> Product1/1, Product2/1, Product3/1
  Product2/1 -> Mux1/4
  Amplitude table lookup4/1 -> Product2/2
  Product3/1 -> Mux1/6
  Amplitude table lookup6/1 -> Product3/2
  psi_r/1 -> "[-inf inf] to [-pi pi]"/1
  U/1 -> Amplitude table lookup1/3, Amplitude table lookup2/3, Amplitude table lookup3/3, Amplitude table lookup4/3, Amplitude table lookup6/3, Phase table lookup1/3, Phase table lookup2/3, Phase table lookup3/3, Phase table lookup4/3, Phase table lookup6/3, Phase table lookup5/3, Amplitude table lookup5/3
  Mux2/1 -> phase/1
  Phase table lookup1/1 -> Mux2/1
  Phase table lookup2/1 -> Mux2/2
  Phase table lookup3/1 -> Mux2/3
  Phase table lookup4/1 -> Mux2/4
  Phase table lookup5/1 -> Mux2/5
  Phase table lookup6/1 -> Mux2/6
  Mux1/1 -> amp/1

== system marine_gnc/Models/Environmental Loads/Utilities/Signal smoothing ==
  Signal in : Inport  OutDataType=sfix(16)  OutScaling=2^0
  Signal rate : Inport  Port=2  OutDataType=sfix(16)  OutScaling=2^0
  -1 : Gain  Gain=-1  ParameterDataType=sfix(16)  ParameterScaling=2^0  OutDataType=sfix(16)  OutScaling=2^0
  Abs : Abs
  Constant : Constant  Value=0  OutDataTypeMode=boolean  OutDataType=sfix(16)  OutScaling=2^0  OutDataTypeStr=boolean
  MinMax Running Resettable : simulink/Math Operations/MinMax Running Resettable  Function=max  vinit=0.0
  Rate Limiter Dynamic : simulink/Discontinuities/Rate Limiter Dynamic
  Signal out : Outport  OutDataType=sfix(16)  OutScaling=2^0
  wires:
  MinMax Running Resettable/1 -> -1/1, Rate Limiter Dynamic/1
  Rate Limiter Dynamic/1 -> Signal out/1
  -1/1 -> Rate Limiter Dynamic/3
  Signal in/1 -> Rate Limiter Dynamic/2
  Constant/1 -> MinMax Running Resettable/2
  Signal rate/1 -> Abs/1
  Abs/1 -> MinMax Running Resettable/1

== system marine_gnc/Models/Environmental Loads/Utilities/Yaw quantizer ==
  psi LF : Inport  OutDataType=sfix(16)  OutScaling=2^0
  psi wave : Inport  Port=2  OutDataType=sfix(16)  OutScaling=2^0
  Backlash : Backlash  BacklashWidth=back
  Quantizer : Quantizer  QuantizationInterval=quant
  Quantizer flag : Constant  Value=quant_flag  OutDataType=sfix(16)  OutScaling=2^0
  Sum : Sum  Inputs=|-+  OutDataType=sfix(16)  OutScaling=2^0
  Switch : Switch  Threshold=0.5
  psi_r quantized : Outport  OutDataType=sfix(16)  OutScaling=2^0
  wires:
  Quantizer flag/1 -> Switch/2
  Switch/1 -> Sum/1
  psi wave/1 -> Sum/2
  Sum/1 -> psi_r quantized/1
  psi LF/1 -> Backlash/1, Switch/3
  Backlash/1 -> Quantizer/1
  Quantizer/1 -> Switch/1
